simulink model "etc_plant_ss"  (R2018a)
settings: Solver=VariableStepAuto  StartTime=0.0  StopTime=20  RelTol=1e-3  EnableMultiTasking=on
PreLoadFcn:
  | etc_plant_data;
values from neighbouring files (symbols this model uses):
  Cs = 3.0    (= 3)    [etc_plant_data.m]    (also in etc_plant_data_limit.m)
  J = 2.4500e-004    (= 0.000245)    [etc_plant_data.m]    (also in etc_plant_data_limit.m)
  Kd = 0.03    [etc_plant_data.m]    (also in etc_plant_data_limit.m)
  Ks = 0.2    [etc_plant_data.m]    (also in etc_plant_data_limit.m)
  theta_eq = pi/6    (= 0.523598775598)    [etc_plant_data.m]    (also in etc_plant_data_limit.m)
settings Model: Creator=nicholas  LastModifiedBy=bneiswan
settings SolverCC: ZeroCrossControl=EnableAll  AutoInsertRateTranBlk=on
settings DataIOCC: ExternalInput=[t, direction, duty]  LoadExternalInput=on  SaveState=on
settings OptimizationCC: ExpressionDepthLimit=2147483647  InitFltsAndDblsToZero=on  LifeSpan=1
settings DebuggingCC: SaveWithParameterizedLinksMsg=none  UnderspecifiedInitializationDetection=Classic  MergeDetectMultiDrivingBlocksExec=none  SignalResolutionControl=TryResolveAllWithWarning  MultiTaskDSMMsg=warning  MultiTaskCondExecSysMsg=none  ParameterPrecisionLossMsg=none  FcnCallInpInsideContextMsg=warning  AllowSymbolicDim=off  StateNameClashWarn=warning  SFUnexpectedBacktrackingDiag=warning  SFNoUnconditionalDefaultTransitionDiag=warning  SFExecutionAtInitializationDiag=none
settings HardwareCC: ProdBitPerPointer=32  ProdBitPerSizeT=32  ProdBitPerPtrDiffT=32  ProdLargestAtomicFloat=None  ProdIntDivRoundTo=Undefined  ProdEndianess=Unspecified  ProdWordSize=32  ProdHWDeviceType=32-bit Generic
settings ModelReferenceCC: PropagateSignalLabelsOutOfModel=off
settings SFSimCC: MATLABDynamicMemAlloc=off
settings RTWCC: SystemTargetFile=ert.tlc  GenCodeOnly=on  TemplateMakefile=ert_default_tmf  Description=RTW Embedded Coder (no auto configuration)
settings CodeAppCC: IgnoreCustomStorageClasses=off  CustomSymbolStrType=$N$R$M  StateflowObjectComments=on  InternalIdentifier=Classic
settings ERTTargetCC: TargetFcnLib=ansi_tfl_tmw.mat  MultiwordLength=2048  GenerateSampleERTMain=on  ERTCustomFileTemplate=example_file_process.tlc  ConvertIfToSwitch=off  SuppressUnreachableDefaultCases=off
settings ConfigComp: CovMetricSettings=dw  CovHtmlReporting=on  CovSaveCumulativeToWorkspaceVar=on  CovSaveSingleToWorkspaceVar=on  CovExternalEMLEnable=off  CovSFcnEnable=off

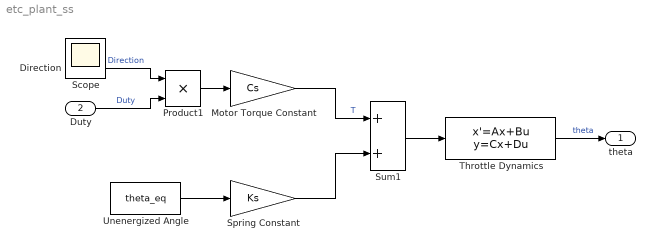
== system etc_plant_ss ==
  Direction : Inport
  Duty : Inport  Port=2
  Motor Torque Constant : Gain  Gain=Cs  SaturateOnIntegerOverflow=on  OutDataTypeStr=Inherit: Same as input  ParamDataTypeStr=Inherit: Same as input
  Product1 : Product  SaturateOnIntegerOverflow=on  OutDataTypeStr=Inherit: Same as first input
  Spring Constant : Gain  Gain=Ks  SaturateOnIntegerOverflow=on  OutDataTypeStr=Inherit: Same as input  ParamDataTypeStr=Inherit: Same as input
  Sum1 : Sum  SaturateOnIntegerOverflow=on
  Throttle Dynamics : StateSpace  A=[0 1;-Ks/J -Kd/J]  B=[0;1/J]  C=[1 0]  D=0  InitialCondition=[pi/6;0]
  Unenergized Angle : Constant  Value=theta_eq
  theta : Outport
  Scope : Scope
  wires:
  Product1/1 -> Motor Torque Constant/1
  Unenergized Angle/1 -> Spring Constant/1
  Direction/1 -> Product1/1  "Direction"
  Duty/1 -> Product1/2  "Duty"
  Motor Torque Constant/1 -> Sum1/1  "T"
  Spring Constant/1 -> Sum1/2
  Sum1/1 -> Throttle Dynamics/1
  Throttle Dynamics/1 -> theta/1  "theta"
